simulink model "Boost_Final"  (R2022b)
settings: Solver=VariableStepAuto  StartTime=0.0  StopTime=1  RelTol=1e-3
libraries: spsDiodeLib x7, spsRMSLib x6, spsSeriesRLCBranchLib x5, spsCurrentMeasurementLib x2, spsVoltageMeasurementLib x2, spsIGBTDiodeLib x1, spsPermanentMagnetSynchronousMachineLib x1, eePowerMeasurement x1, spsThreePhaseVIMeasurementLib x1, spsWindTurbineLib x1, spspowerguiLib x1
settings Model: Creator=NITISH AGGARWAL  LastModifiedBy=shubh
settings DebuggingCC: UnconnectedInputMsg=warning  UnconnectedOutputMsg=warning  UnconnectedLineMsg=warning
settings ModelReferenceCC: EnableRefExpFcnMdlSchedulingChecks=on
settings RTWCC: DLArmComputeVersion=19.05

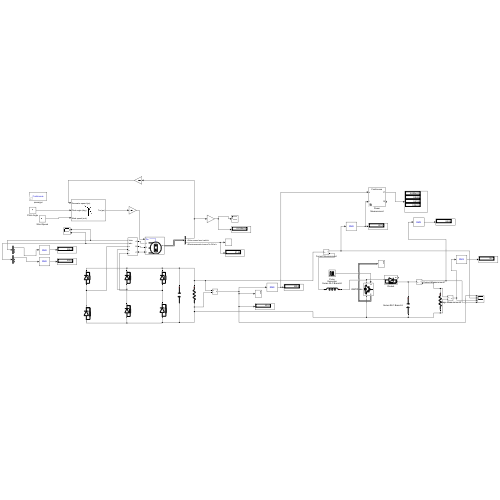
[thumbnail: Simulink's stored preview of the top-level diagram]
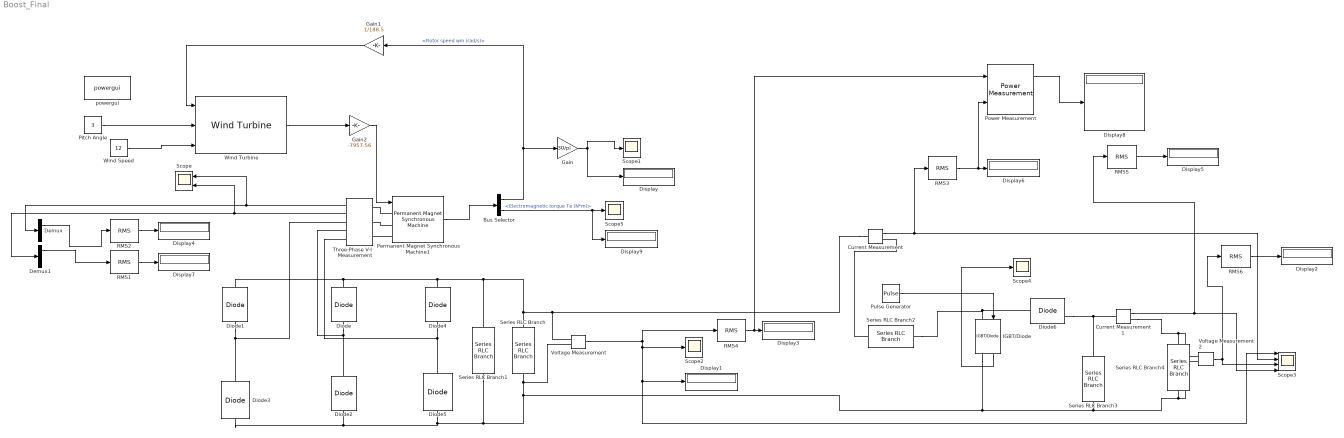
== system Boost_Final ==
  Bus Selector : BusSelector  OutputSignals=Rotor speed wm (rad/s),Electromagnetic torque Te (N*m)
  Current Measurement : spsCurrentMeasurementLib/Current Measurement  PhasorSimulation=off  OutputType=Complex  PSBequivalent=0
  Current Measurement1 : spsCurrentMeasurementLib/Current Measurement  PhasorSimulation=off  OutputType=Complex  PSBequivalent=0
  Demux : Demux  Outputs=3
  Demux1 : Demux  Outputs=3
  Diode{,1..5} (6 alike) : spsDiodeLib/Diode  Ron=0.001  Lon=0  Vf=0.8  IC=0  UseSnubber=0  Rs=500  Cs=250e-9  Measurements=off
  Diode6 : spsDiodeLib/Diode  Ron=0.001  Lon=0  Vf=0.8  IC=0  UseSnubber=0  Rs=500  Cs=250e-9  Measurements=on
  Display{,1..9} (10 alike) : Display
  Gain : Gain  Gain=30/pi
  Gain1 : Gain  Gain=1/188.5
  Gain2 : Gain  Gain=-7957.56
  IGBT/Diode : spsIGBTDiodeLib/IGBT//Diode  Ron=1e-3  Rs=1e5  Cs=inf  Measurements=on
  Permanent Magnet Synchronous Machine1 : spsPermanentMagnetSynchronousMachineLib/Permanent Magnet Synchronous Machine  NbPhases=3  FluxDistribution=Sinusoidal  RotorType=Round  MechanicalLoad=Torque Tm  PresetModel=No  ShowDetailedParameters=on  MeasurementBus=off  Resistance=0.0485  Inductance=8.5e-3  dqInductances=[8.5e-3,8.5e-3]  La=0.000395  MachineConstant=Flux linkage established by magnets (V.s)  Flux=0.1194  VoltageCst=86.6271  TorqueCst=0.7164  Flat=120  Mechanical=[0.0027 0.0004924 4 0]  PolePairs=4  InitialConditions=[0,0, 0,0]  InitialConditions5ph=[0 0 0 0 0 0]  RefAngle=90 degrees behind phase A axis (modified Park)  IterativeDiscreteModel=Trapezoidal non iterative  TsBlock=-1  TsPowergui=0
  Pitch Angle : Constant  Value=3
  Power Measurement : eePowerMeasurement/Power Measurement  LabelModeActiveChoice=Continuous  F=60  K=[0 1 2 3]  Ts=0
  Pulse Generator : DiscretePulseGenerator  PulseType=Time based  Amplitude=4  Period=1/5000  PulseWidth=60
  RMS1 : spsRMSLib/RMS  TrueRMS=on  Freq=60  RMSInit=0  Ts=0
  RMS2 : spsRMSLib/RMS  TrueRMS=on  Freq=60  RMSInit=0  Ts=0
  RMS{3..6} (4 alike) : spsRMSLib/RMS  TrueRMS=on  Freq=60  RMSInit=120  Ts=0
  Scope : Scope  NumInputPorts=2
  Scope{1..2,4..5} (4 alike) : Scope
  Scope3 : Scope  NumInputPorts=4
  Series RLC Branch : spsSeriesRLCBranchLib/Series RLC Branch  LConnTagsString=__new0  RConnTagsString=__new0  BranchType=R  Resistance=10  Inductance=1e-3  SetiL0=off  InitialCurrent=0  Capacitance=1e-6  Setx0=off  InitialVoltage=0  Measurements=None
  Series RLC Branch1 : spsSeriesRLCBranchLib/Series RLC Branch  LConnTagsString=__new0  RConnTagsString=__new0  BranchType=C  Resistance=10  Inductance=10e-3  SetiL0=off  InitialCurrent=0  Capacitance=10e-3  Setx0=off  InitialVoltage=0  Measurements=None
  Series RLC Branch2 : spsSeriesRLCBranchLib/Series RLC Branch  LConnTagsString=__new0  RConnTagsString=__new0  BranchType=L  Resistance=1  Inductance=6e-3  SetiL0=off  InitialCurrent=0  Capacitance=1e-6  Setx0=off  InitialVoltage=0  Measurements=None
  Series RLC Branch3 : spsSeriesRLCBranchLib/Series RLC Branch  LConnTagsString=__new0  RConnTagsString=__new0  BranchType=C  Resistance=1  Inductance=6e-3  SetiL0=off  InitialCurrent=0  Capacitance=5000e-6  Setx0=off  InitialVoltage=0  Measurements=None
  Series RLC Branch4 : spsSeriesRLCBranchLib/Series RLC Branch  LConnTagsString=__new0  RConnTagsString=__new0  BranchType=R  Resistance=12.5  Inductance=6e-3  SetiL0=off  InitialCurrent=0  Capacitance=1e-6  Setx0=off  InitialVoltage=0  Measurements=None
  Three-Phase V-I Measurement : spsThreePhaseVIMeasurementLib/Three-Phase V-I Measurement  VoltageMeasurement=phase-to-phase  SetLabelV=off  LabelV=Vabc  Vpu=off  VpuLL=off  CurrentMeasurement=yes  SetLabelI=off  LabelI=Iabc  Ipu=off  Pbase=100e6  Vbase=500e3  OutputType=Complex  PhasorSimulation=off  PSBequivalent=0
  Voltage Measurement : spsVoltageMeasurementLib/Voltage Measurement  PhasorSimulation=off  OutputType=Complex  PSBequivalent=0
  Voltage Measurement2 : spsVoltageMeasurementLib/Voltage Measurement  PhasorSimulation=off  OutputType=Complex  PSBequivalent=0
  Wind Speed : Constant  Value=12
  Wind Turbine : spsWindTurbineLib/Wind Turbine  Pnom=1.5e6  Pelec_base=1.5e6/0.9  wind_base=12  P_wind_base=1  speed_nom=1.2  pitch_angle=0  c1_c6="[0.51763          116          0.4            5           21     0.006795]"  cp_nom=0.48  lambda_nom=8.1
  powergui : spspowerguiLib/powergui  Priority=1  SimulationMode=Continuous  SampleTime=50e-6  frequency=60  Iterations=50  frequencyindice=0  Pbase=100e6  ErrMax=1e-4  UnitsV=kV  UnitsW=MW  buscounter=0  FunctionMessages=off  echomessages=off  EnableUseOfTLC=off  CurrentSourceSwitches=off  DisableSnubberDevices=off  DisableRonSwitches=off  DisableVfSwitches=off  DisplayEquations=off  AutomaticDiscreteSolvers=off  SolverType=Tustin/Backward Euler (TBE)  Interpol=off  ExternalGateDelay=off  methode=off  Ts=100  x0status=blocks  SPID=on  SwTol=0  HookPort=off  NonlinearTolerance=1e-4  nMaxIteration=100  ContinueOnMaxIteration=off  RestoreLinks=warning  ResistiveCurrentMeasurement=off  Frange=[0:2:500]  Ylog=off  Xlog=on  ShowGrid=off  save=off  variable=ZData  structure=0  ZoomFFT=off  StartTime=0.0  cycles=1  DisplayStyle=1  fundamental=60  FreqAxis=off  MaxFrequency=1000  frequencyindicesteady=1  RmsSteady=1  display=off
  wires:
  Wind Speed/1 -> Wind Turbine/3
  Pitch Angle/1 -> Wind Turbine/2
  Permanent Magnet Synchronous Machine1/1 -> Bus Selector/1
  Bus Selector/1 -> Gain1/1, Gain/1  "<Rotor speed wm (rad/s)>"
  Gain/1 -> Display/1, Scope1/1
  IGBT/Diode/1 -> Scope4/1
  Current Measurement1/1 -> RMS5/1, Scope3/4
  RMS6/1 -> Display2/1
  Pulse Generator/1 -> IGBT/Diode/1
  Voltage Measurement2/1 -> RMS6/1, Scope3/3
  Current Measurement/1 -> RMS3/1, Scope3/2
  RMS2/1 -> Display4/1
  Gain1/1 -> Wind Turbine/1
  Wind Turbine/1 -> Gain2/1
  Gain2/1 -> Permanent Magnet Synchronous Machine1/1
  RMS5/1 -> Display5/1
  Voltage Measurement/1 -> RMS4/1, Scope3/1, Display1/1, Scope2/1
  RMS3/1 -> Power Measurement/2, Display6/1
  Three-Phase V-I Measurement/1 -> Demux/1, Scope/1
  Three-Phase V-I Measurement/2 -> Demux1/1, Scope/2
  RMS1/1 -> Display7/1
  RMS4/1 -> Power Measurement/1, Display3/1
  Demux/1 -> RMS2/1
  Demux1/1 -> RMS1/1
  Power Measurement/1 -> Display8/1
  Bus Selector/2 -> Display9/1, Scope5/1  "<Electromagnetic torque Te (N*m)>"
  connections:
  Permanent Magnet Synchronous Machine1/LConn1 -- Three-Phase V-I Measurement/LConn1
  Permanent Magnet Synchronous Machine1/LConn2 -- Three-Phase V-I Measurement/LConn2
  Permanent Magnet Synchronous Machine1/LConn3 -- Three-Phase V-I Measurement/LConn3
  Diode1/LConn1 -- Three-Phase V-I Measurement/RConn1 -- Diode3/RConn1
  Diode/LConn1 -- Three-Phase V-I Measurement/RConn2 -- Diode2/RConn1
  Diode4/LConn1 -- Three-Phase V-I Measurement/RConn3 -- Diode5/RConn1
  IGBT/Diode/RConn1 -- Voltage Measurement2/LConn2 -- Series RLC Branch4/RConn1 -- Series RLC Branch3/RConn1 -- Voltage Measurement/LConn2 -- Series RLC Branch/RConn1 -- Series RLC Branch1/RConn1 -- Diode5/LConn1 -- Diode3/LConn1 -- Diode2/LConn1
  Current Measurement/LConn1 -- Voltage Measurement/LConn1 -- Series RLC Branch/LConn1 -- Series RLC Branch1/LConn1 -- Diode1/RConn1 -- Diode/RConn1 -- Diode4/RConn1
  Diode6/RConn1 -- Series RLC Branch3/LConn1 -- Current Measurement1/LConn1
  Series RLC Branch2/LConn1 -- IGBT/Diode/LConn1 -- Diode6/LConn1
  Voltage Measurement2/LConn1 -- Current Measurement1/RConn1 -- Series RLC Branch4/LConn1
  Series RLC Branch2/RConn1 -- Current Measurement/RConn1
